simulink model "torqueControlBalancingR2022a"  (R2022a)
settings: Solver=FixedStepDiscrete  StartTime=0.0  StopTime=Config.SIMULATION_TIME  FixedStep=Config.tStep  RelTol=1e-3  EnableMultiTasking=on
PostLoadFcn:
  | %% Try to open the static GUI and try to adjust it
  | try
  | 
  |     staticGUI = simulinkStaticGUI;
  | 
  | end
InitFcn:
  | %% initialize the simulation
  | cd(fileparts(which(bdroot)));
  | initTorqueControlBalancing;
  | 
  | %% Try to edit the GUI (the user may have already closed it)
  | try
  | 
  |     %% Update Start Button
  |     set(sl_synch_handles.startButton,'Backgroundcolor',[0.0,1.0,0.0]);
  |     set(sl_synch_handles.startButton,'Enable','on');
  | 
  | end
StartFcn:
  | %% Try to edit the GUI (the user may have already closed it)
  | try
  | 
  |     %% Update Start Button
  |     set(sl_synch_handles.startButton,'Backgroundcolor',[0.8,0.8,0.8]);
  |     set(sl_synch_handles.startButton,'Enable','off');
  | 
  |     %% Update Compile Button
  |     set(sl_synch_handles.compileButton,'Backgroundcolor',[0.8,0.8,0.8]);
  |     set(sl_synch_handles.compileButton,'Enable','off');
  | 
  |     %% Update Exit Button
  |     set(sl_synch_handles.exitButton,'Backgroundcolor',[0.8,0.8,0.8]);
  |     set(sl_synch_handles.exitButton,'Enable','off');
  | 
  | end
StopFcn:
  | %% stop the simulation
  | cd(fileparts(which(bdroot)));
  | stopTorqueControlBalancing;
  | 
  | %% Try to edit the GUI (the user may have already closed it)
  | try
  | 
  |     %% Update Start Button
  |     if get(sl_synch_handles.checkbox_recompile, 'Value')
  |         set(sl_synch_handles.startButton,'Backgroundcolor',[0.0,1.0,0.0]);
  |         set(sl_synch_handles.startButton,'Enable','on');
  |     end
  | 
  |     %% Update Compile Button
  |     set(sl_synch_handles.compileButton,'Backgroundcolor',[1.0,0.6,0.0]);
  |     set(sl_synch_handles.compileButton,'Enable','on');
  | 
  |     %% Update Exit Button
  |     set(sl_synch_handles.exitButton,'Backgroundcolor',[0.0,1.0,1.0]);
  |     set(sl_synch_handles.exitButton,'Enable','on');
  | 
  | end
undefined symbols (not defined in the file or in its folder): bVectorConstraints, Config, ConstraintsMatrix, Gain, Reg, ROBOT_DOF, Sat, StateMachine
libraries: WBToolboxLibrary x57
(part 1 of 2)
CloseFcn:
  | %% Try to close the GUI (the user might have already closed it)
  | try
  | 
  |     close(simulinkStaticGUI)
  | 
  | end
settings Model: Creator=daniele  LastModifiedBy=dpucci
settings SolverCC: AlgebraicLoopSolver=TrustRegion
settings DataIOCC: LimitDataPoints=on  SaveFormat=Array  ReturnWorkspaceOutputs=off
settings OptimizationCC: ExpressionDepthLimit=2147483647  ZeroExternalMemoryAtStartup=off  ZeroInternalMemoryAtStartup=off  LifeSpan=inf
settings DebuggingCC: UnderspecifiedInitializationDetection=Classic  MergeDetectMultiDrivingBlocksExec=none  SolverPrmCheckMsg=warning  FcnCallInpInsideContextMsg=warning  UnconnectedInputMsg=warning  UnconnectedOutputMsg=warning  UnconnectedLineMsg=warning  AllowSymbolicDim=off  StateNameClashWarn=warning  SFUnexpectedBacktrackingDiag=warning  SFNoUnconditionalDefaultTransitionDiag=warning  SFExecutionAtInitializationDiag=none  ArithmeticOperatorsInVariantConditions=warning
settings HardwareCC: ProdBitPerPointer=32  ProdBitPerSizeT=32  ProdBitPerPtrDiffT=32  ProdLargestAtomicFloat=None  ProdIntDivRoundTo=Undefined  ProdEndianess=Unspecified  ProdWordSize=32  ProdHWDeviceType=32-bit Generic
settings ModelReferenceCC: PropagateSignalLabelsOutOfModel=off
settings SFSimCC: SimUseLocalCustomCode=off  SimParseCustomCode=off  CustomCodeUndefinedFunction=UseInterfaceOnly  SimTargetLang=C++
settings RTWCC: GenCodeOnly=on  RTWUseLocalCustomCode=off  TargetLang=C++
settings CodeAppCC: StateflowObjectComments=on
settings GRTTargetCC: TargetLangStandard=C++03 (ISO)  MatFileLogging=off  CodeInterfacePackaging=C++ class  SupportNonFinite=off
settings ConfigComp: CovMetricSettings=dw  CovSaveCumulativeToWorkspaceVar=on  CovSaveSingleToWorkspaceVar=on  CovExternalEMLEnable=off

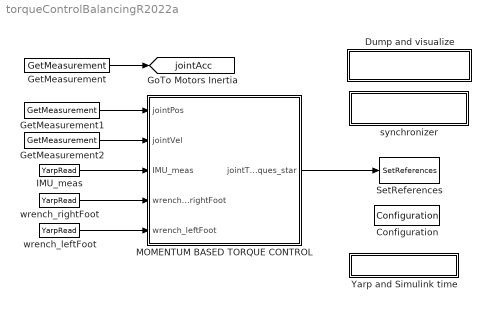
== system torqueControlBalancingR2022a ==
  " Yarp and Simulink time" : Subsystem
  Configuration : WBToolboxLibrary/Utilities/Configuration  ConfigSource=Workspace  ConfigObject='WBTConfigRobot'  RobotName='icubSim'  UrdfFile='model.urdf'  ControlledJoints={'l_elbow','l_shoulder_pitch','torso_roll'}  ControlBoardsNames={'left_arm','right_arm','torso'}  LocalName='WBT'  GravityVector=[0,0,-9.81]
      settings: SourceProductName=WholeBodyToolbox
  Dump and visualize : Subsystem
      mask Display: disp('VISUALIZER')
  GetMeasurement : WBToolboxLibrary/States/GetMeasurement  measuredType=Joints Acceleration
      settings: SourceProductName=WholeBodyToolbox
  GetMeasurement1 : WBToolboxLibrary/States/GetMeasurement  measuredType=Joints Position
      settings: SourceProductName=WholeBodyToolbox
  GetMeasurement2 : WBToolboxLibrary/States/GetMeasurement  measuredType=Joints Velocity
      settings: SourceProductName=WholeBodyToolbox
  IMU_meas : WBToolboxLibrary/Utilities/YarpRead  portName=Ports.IMU  signalSize=Ports.IMU_PORT_SIZE  timeout=0.5  blocking=off  timestamp=off  autoconnect=on  errorOnConnection=off
      settings: SourceProductName=WholeBodyToolbox
  MOMENTUM BASED TORQUE CONTROL : Subsystem
  SetReferences : WBToolboxLibrary/Actuators/SetReferences  controlType=Torque  refSpeed=50  refAcceleration=1000000*(pi/180)
      settings: SourceProductName=WholeBodyToolbox
  synchronizer : Subsystem
      mask Display: disp('SYNCHRONIZER')
  wrench_leftFoot : WBToolboxLibrary/Utilities/YarpRead  portName=Ports.WRENCH_LEFT_FOOT  signalSize=Ports.WRENCH_PORT_SIZE  timeout=0.5  blocking=off  timestamp=off  autoconnect=on  errorOnConnection=on
      settings: SourceProductName=WholeBodyToolbox
  wrench_rightFoot : WBToolboxLibrary/Utilities/YarpRead  portName=Ports.WRENCH_RIGHT_FOOT  signalSize=Ports.WRENCH_PORT_SIZE  timeout=0.5  blocking=off  timestamp=off  autoconnect=on  errorOnConnection=on
      settings: SourceProductName=WholeBodyToolbox
  tag scope: jointAcc=global
  wires:
  MOMENTUM BASED TORQUE CONTROL/1(jointTorques_star) -> SetReferences/1
  GetMeasurement/1 -> [jointAcc]
  GetMeasurement2/1 -> MOMENTUM BASED TORQUE CONTROL/2(jointVel)
  GetMeasurement1/1 -> MOMENTUM BASED TORQUE CONTROL/1(jointPos)
  IMU_meas/1 -> MOMENTUM BASED TORQUE CONTROL/3(IMU_meas)
  wrench_rightFoot/1 -> MOMENTUM BASED TORQUE CONTROL/4(wrench_rightFoot)
  wrench_leftFoot/1 -> MOMENTUM BASED TORQUE CONTROL/5(wrench_leftFoot)

== system torqueControlBalancingR2022a/ Yarp and Simulink time ==
  Clock : Clock
  Sum : Sum  Inputs=+-|
  Sum1 : Sum  Inputs=|+-
  Yarp Clock : WBToolboxLibrary/Utilities/Yarp Clock
      settings: SourceProductName=WholeBodyToolbox
  "holder " : WBToolboxLibrary/Utilities/holder 
      settings: SourceProductName=WholeBodyToolbox
  time : Scope  NumInputPorts=3
  wires:
  Yarp Clock/1 -> "holder "/1, Sum1/1  "Yarp-time"
  Sum/1 -> time/3  "Difference Simulink - Yarp time"
  Sum1/1 -> Sum/2, time/2  "Yarp-time_0"
  "holder "/1 -> Sum1/2
  Clock/1 -> Sum/1, time/1  "Simulink-time"

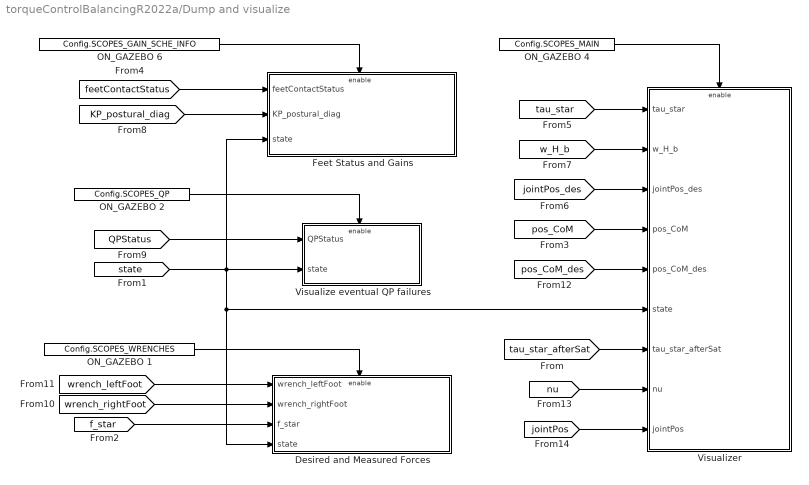
== system torqueControlBalancingR2022a/Dump and visualize ==
  Desired and Measured Forces : Subsystem
  Feet Status and Gains : Subsystem
  ON_GAZEBO 1 : Constant  Value=Config.SCOPES_WRENCHES
  ON_GAZEBO 2 : Constant  Value=Config.SCOPES_QP
  ON_GAZEBO 4 : Constant  Value=Config.SCOPES_MAIN
  ON_GAZEBO 6 : Constant  Value=Config.SCOPES_GAIN_SCHE_INFO
  Visualize eventual QP failures : Subsystem
  Visualizer : Subsystem
  wires:
  ON_GAZEBO 4/1 -> Visualizer/Enable
  [state] -> Visualize eventual QP failures/2(state), Desired and Measured Forces/4(state), Visualizer/6(state), Feet Status and Gains/3(state)
  [w_H_b] -> Visualizer/2(w_H_b)
  [tau_star] -> Visualizer/1(tau_star)
  [pos_CoM_des] -> Visualizer/5(pos_CoM_des)
  ON_GAZEBO 2/1 -> Visualize eventual QP failures/Enable
  [QPStatus] -> Visualize eventual QP failures/1(QPStatus)
  ON_GAZEBO 1/1 -> Desired and Measured Forces/Enable
  ON_GAZEBO 6/1 -> Feet Status and Gains/Enable
  [feetContactStatus] -> Feet Status and Gains/1(feetContactStatus)
  [KP_postural_diag] -> Feet Status and Gains/2(KP_postural_diag)
  [f_star] -> Desired and Measured Forces/3(f_star)
  [wrench_leftFoot] -> Desired and Measured Forces/1(wrench_leftFoot)
  [wrench_rightFoot] -> Desired and Measured Forces/2(wrench_rightFoot)
  [jointPos_des] -> Visualizer/3(jointPos_des)
  [pos_CoM] -> Visualizer/4(pos_CoM)
  [tau_star_afterSat] -> Visualizer/7(tau_star_afterSat)
  [nu] -> Visualizer/8(nu)
  [jointPos] -> Visualizer/9(jointPos)

== system torqueControlBalancingR2022a/MOMENTUM BASED TORQUE CONTROL ==
  jointPos : Inport
  jointVel : Inport  Port=2
  IMU_meas : Inport  Port=3
  wrench_rightFoot : Inport  Port=4
  wrench_leftFoot : Inport  Port=5
  Balancing Controller QP : Subsystem
  Dynamics and Kinematics : Subsystem
  Joint Torque Saturation : Subsystem
  Robot State and References : Subsystem  Priority=-10
  emergency stop: joint limits : Subsystem
      mask Display: disp('EMERGENCY STOP')
  jointTorques_star : Outport  VectorParamsAs1DForOutWhenUnconnected=off
  wires:
  Dynamics and Kinematics/4(w_H_l_sole) -> Balancing Controller QP/4(w_H_l_sole)
  Dynamics and Kinematics/11(JDot_r_sole_nu) -> Balancing Controller QP/11(JDot_r_sole_nu)
  Dynamics and Kinematics/9(pos_CoM) -> Balancing Controller QP/9(pos_CoM)
  Dynamics and Kinematics/2(h) -> Balancing Controller QP/2(h)
  Dynamics and Kinematics/8(J_CoM) -> Balancing Controller QP/8(J_CoM)
  Dynamics and Kinematics/5(w_H_r_sole) -> Balancing Controller QP/5(w_H_r_sole)
  Robot State and References/2(nu) -> Balancing Controller QP/13(nu), Dynamics and Kinematics/2(nu)
  Robot State and References/7(KD_CoM) -> Balancing Controller QP/18(KD_CoM)
  jointVel/1 -> Robot State and References/2(jointVel)
  Joint Torque Saturation/1(tau_star_sat) -> jointTorques_star/1
  Dynamics and Kinematics/7(J_r_sole) -> Balancing Controller QP/7(J_r_sole)
  Robot State and References/3(state) -> Balancing Controller QP/14(state)
  Balancing Controller QP/1("tau_star ") -> Joint Torque Saturation/1(tau_star)
  Dynamics and Kinematics/6(J_l_sole) -> Balancing Controller QP/6(J_l_sole)
  Dynamics and Kinematics/1(M) -> Balancing Controller QP/1(M)
  Robot State and References/6(KP_CoM) -> Balancing Controller QP/17(KP_CoM)
  Dynamics and Kinematics/3(L) -> Balancing Controller QP/3("L ")
  Robot State and References/9(jointPos_des) -> Balancing Controller QP/20(jointPos_des)
  Robot State and References/4(feetContactStatus) -> Balancing Controller QP/15(feetContactStatus)
  IMU_meas/1 -> Robot State and References/3(IMU_meas)
  Robot State and References/1(w_H_b) -> Dynamics and Kinematics/1(w_H_b)
  Robot State and References/5(KP_postural) -> Balancing Controller QP/16(KP_postural)
  Dynamics and Kinematics/10(JDot_l_sole_nu) -> Balancing Controller QP/10(JDot_l_sole_nu)
  Robot State and References/8(desired_pos_vel_acc_CoM) -> Balancing Controller QP/19(desired_pos_vel_acc_CoM)
  jointPos/1 -> emergency stop: joint limits/1(jointPos), Robot State and References/1(jointPos), Dynamics and Kinematics/3(jointPos), Balancing Controller QP/12(jointPos)
  wrench_rightFoot/1 -> Robot State and References/4(wrench_rightFoot)
  wrench_leftFoot/1 -> Robot State and References/5(wrench_leftFoot)

== system torqueControlBalancingR2022a/synchronizer ==
  GAZEBO_SYNCHRONIZER : Subsystem
  Logical Operator : Logic  Operator=NOT  AllPortsSameDT=off  OutDataTypeStr=boolean
  "ON_GAZEBO " : Constant  Value=Config.ON_GAZEBO
  REAL_TIME_SYNC : Subsystem
  To Workspace : ToWorkspace  VariableName=yarp_time  SaveFormat=Structure With Time  SampleTime=-1
  Yarp Clock : WBToolboxLibrary/Utilities/Yarp Clock
      settings: SourceProductName=WholeBodyToolbox
  wires:
  Logical Operator/1 -> REAL_TIME_SYNC/Enable
  "ON_GAZEBO "/1 -> GAZEBO_SYNCHRONIZER/Enable, Logical Operator/1
  Yarp Clock/1 -> To Workspace/1

== system torqueControlBalancingR2022a/Dump and visualize/Desired and Measured Forces ==
  wrench_leftFoot : Inport
  wrench_rightFoot : Inport  Port=2
  f_star : Inport  Port=3
  state : Inport  Port=4
  Enable : EnablePort
  Constant : Constant  Value=StateMachine.wrench_thresholdContactOn
  Constant2 : Constant  Value=StateMachine.wrench_thresholdContactOff
  Demux Forces nd Moments : Subsystem
  Sum{,1..3} (4 alike) : Sum  Inputs=-+|
  left Foot forces : Scope  NumInputPorts=6
  left Foot moments : Scope  NumInputPorts=4
  right Foot forces : Scope  NumInputPorts=6
  right Foot moments : Scope  NumInputPorts=4
  wires:
  wrench_leftFoot/1 -> Demux Forces nd Moments/1(wrench_leftFoot)
  wrench_rightFoot/1 -> Demux Forces nd Moments/2(wrench_rightFoot)
  f_star/1 -> Demux Forces nd Moments/3(f_star)
  Demux Forces nd Moments/1(measured forces l_sole) -> left Foot forces/1, Sum/1  "measured forces l_sole"
  Demux Forces nd Moments/2(des forces l_sole) -> Sum/2, left Foot forces/2  "desired forces l_sole"
  Sum/1 -> left Foot forces/3  "error forces l_sole"
  Constant/1 -> right Foot forces/5, left Foot forces/5  "thresholdContactOn"
  Demux Forces nd Moments/4(des forces r_sole) -> Sum1/2, right Foot forces/2  "desired forces r_sole"
  Demux Forces nd Moments/3(measured forces r_sole) -> right Foot forces/1, Sum1/1  "measured forces r_sole"
  Sum1/1 -> right Foot forces/3  "error forces r_sole"
  Constant2/1 -> left Foot forces/4, right Foot forces/4  "thresholdContactOff"
  Demux Forces nd Moments/7(measured moments r_sole) -> Sum3/1, right Foot moments/1  "measured moments r_sole"
  state/1 -> right Foot moments/4, left Foot moments/4, right Foot forces/6, left Foot forces/6  "state"
  Demux Forces nd Moments/8(des moments r_sole) -> right Foot moments/2, Sum3/2  "desired moments r_sole"
  Sum3/1 -> right Foot moments/3  "error moments r_sole"
  Sum2/1 -> left Foot moments/3  "error moments l_sole"
  Demux Forces nd Moments/6(des moments l_sole) -> Sum2/2, left Foot moments/2  "desired moments l_sole"
  Demux Forces nd Moments/5(measured moments l_sole) -> Sum2/1, left Foot moments/1  "measured moments l_sole"

== system torqueControlBalancingR2022a/Dump and visualize/Feet Status and Gains ==
  feetContactStatus : Inport
  KP_postural_diag : Inport  Port=2
  state : Inport  Port=3
  Enable : EnablePort
  Demux1 : Demux  Outputs=Config.numOfJointsForEachControlboard
  Feet Contact Activation : Scope  NumInputPorts=2
  Gain Scheduling Postural : Scope  NumInputPorts=6
  wires:
  state/1 -> Feet Contact Activation/2, Gain Scheduling Postural/6
  feetContactStatus/1 -> Feet Contact Activation/1
  KP_postural_diag/1 -> Demux1/1
  Demux1/4 -> Gain Scheduling Postural/4  "left_leg"
  Demux1/5 -> Gain Scheduling Postural/5  "right_leg"
  Demux1/3 -> Gain Scheduling Postural/3  "right_arm"
  Demux1/1 -> Gain Scheduling Postural/1  "torso"
  Demux1/2 -> Gain Scheduling Postural/2  "left_arm"

== system torqueControlBalancingR2022a/Dump and visualize/Visualize eventual QP failures ==
  QPStatus : Inport
  state : Inport  Port=2
  Enable : EnablePort
  QP status (0: no failure) : Scope  NumInputPorts=2
  wires:
  QPStatus/1 -> QP status (0: no failure)/1
  state/1 -> QP status (0: no failure)/2

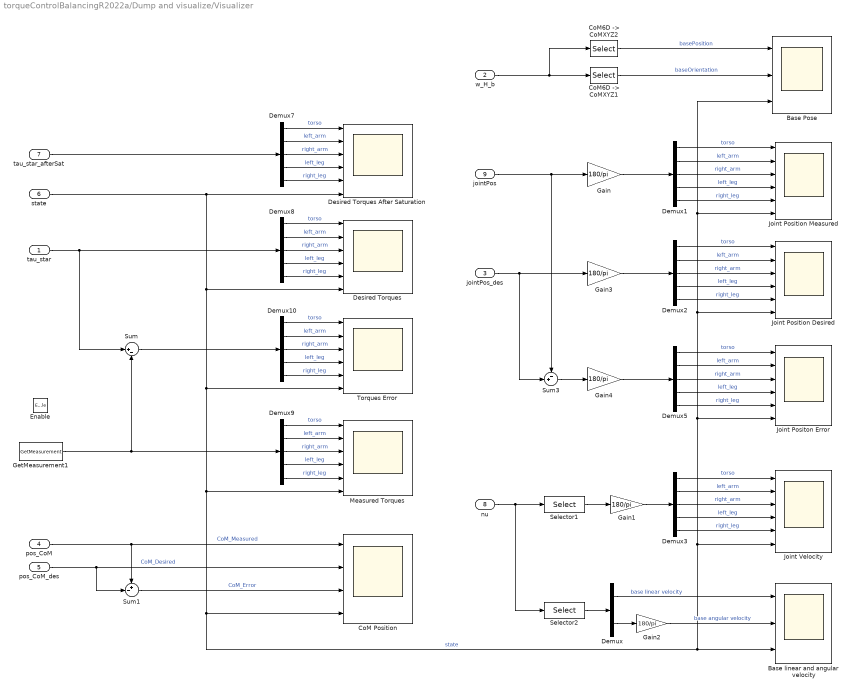
== system torqueControlBalancingR2022a/Dump and visualize/Visualizer ==
  tau_star : Inport
  w_H_b : Inport  Port=2
  jointPos_des : Inport  Port=3
  pos_CoM : Inport  Port=4
  pos_CoM_des : Inport  Port=5
  state : Inport  Port=6
  tau_star_afterSat : Inport  Port=7
  nu : Inport  Port=8
  jointPos : Inport  Port=9
  Enable : EnablePort
  Base Pose : Scope  NumInputPorts=3
  Base linear and angular velocity : Scope  NumInputPorts=3
  CoM Position : Scope  NumInputPorts=4
  "CoM6D -> CoMXYZ1" : Selector  NumberOfDimensions=2  InputPortWidth=7  IndexOptions=Index vector (dialog),Index vector (dialog)  Indices=[1 2 3],[1 2 3]  OutputSizes=1,1
  "CoM6D -> CoMXYZ2" : Selector  NumberOfDimensions=2  InputPortWidth=7  IndexOptions=Index vector (dialog),Index vector (dialog)  Indices=[1 2 3],[4]  OutputSizes=1,1
  Demux : Demux  Outputs=2
  Demux{1..3,5,7..10} (8 alike) : Demux  Outputs=Config.numOfJointsForEachControlboard
  Desired Torques : Scope  NumInputPorts=6
  Desired Torques After Saturation : Scope  NumInputPorts=6
  Gain{,1..4} (5 alike) : Gain  Gain=180/pi
  GetMeasurement1 : WBToolboxLibrary/States/GetMeasurement  measuredType=Joints Torque
      settings: SourceProductName=WholeBodyToolbox
  Joint Position Desired : Scope  NumInputPorts=6
  Joint Position Measured : Scope  NumInputPorts=6
  Joint Positon Error : Scope  NumInputPorts=6
  Joint Velocity : Scope  NumInputPorts=6
  Measured Torques : Scope  NumInputPorts=6
  Selector1 : Selector  InputPortWidth=6+ROBOT_DOF  IndexOptions=Index vector (dialog)  Indices=[7:6+ROBOT_DOF]  OutputSizes=1
  Selector2 : Selector  InputPortWidth=6+ROBOT_DOF  IndexOptions=Index vector (dialog)  Indices=[1:6]  OutputSizes=1
  Sum : Sum  Inputs=|+-
  Sum1 : Sum  Inputs=+-|
  Sum3 : Sum  Inputs=-+|
  Torques Error : Scope  NumInputPorts=6
  wires:
  pos_CoM/1 -> Sum1/1, CoM Position/1  "CoM_Measured"
  Gain/1 -> Demux1/1
  jointPos/1 -> Gain/1, Sum3/1
  Demux1/5 -> Joint Position Measured/5  "right_leg"
  Demux1/1 -> Joint Position Measured/1  "torso"
  Demux1/2 -> Joint Position Measured/2  "left_arm"
  Demux1/4 -> Joint Position Measured/4  "left_leg"
  Demux1/3 -> Joint Position Measured/3  "right_arm"
  GetMeasurement1/1 -> Sum/2, Demux9/1
  Demux8/5 -> Desired Torques/5  "right_leg"
  Demux8/1 -> Desired Torques/1  "torso"
  Demux8/2 -> Desired Torques/2  "left_arm"
  Demux8/4 -> Desired Torques/4  "left_leg"
  Demux8/3 -> Desired Torques/3  "right_arm"
  Demux10/5 -> Torques Error/5  "right_leg"
  Demux10/1 -> Torques Error/1  "torso"
  Demux10/2 -> Torques Error/2  "left_arm"
  Demux10/4 -> Torques Error/4  "left_leg"
  Demux10/3 -> Torques Error/3  "right_arm"
  Sum/1 -> Demux10/1
  Demux9/5 -> Measured Torques/5  "right_leg"
  Demux9/1 -> Measured Torques/1  "torso"
  Demux9/2 -> Measured Torques/2  "left_arm"
  Demux9/4 -> Measured Torques/4  "left_leg"
  Demux9/3 -> Measured Torques/3  "right_arm"
  jointPos_des/1 -> Sum3/2, Gain3/1
  Gain3/1 -> Demux2/1
  Demux2/5 -> Joint Position Desired/5  "right_leg"
  Demux2/1 -> Joint Position Desired/1  "torso"
  Demux2/2 -> Joint Position Desired/2  "left_arm"
  Demux2/4 -> Joint Position Desired/4  "left_leg"
  Demux2/3 -> Joint Position Desired/3  "right_arm"
  Gain4/1 -> Demux5/1
  Demux5/5 -> Joint Positon Error/5  "right_leg"
  Demux5/1 -> Joint Positon Error/1  "torso"
  Demux5/2 -> Joint Positon Error/2  "left_arm"
  Demux5/4 -> Joint Positon Error/4  "left_leg"
  Demux5/3 -> Joint Positon Error/3  "right_arm"
  Sum3/1 -> Gain4/1
  pos_CoM_des/1 -> Sum1/2, CoM Position/2  "CoM_Desired"
  w_H_b/1 -> "CoM6D -> CoMXYZ2"/1, "CoM6D -> CoMXYZ1"/1
  "CoM6D -> CoMXYZ2"/1 -> Base Pose/1  "basePosition"
  "CoM6D -> CoMXYZ1"/1 -> Base Pose/2  "baseOrientation"
  Demux7/4 -> Desired Torques After Saturation/4  "left_leg"
  Demux7/5 -> Desired Torques After Saturation/5  "right_leg"
  Demux7/2 -> Desired Torques After Saturation/2  "left_arm"
  Demux7/1 -> Desired Torques After Saturation/1  "torso"
  Demux7/3 -> Desired Torques After Saturation/3  "right_arm"
  tau_star_afterSat/1 -> Demux7/1
  tau_star/1 -> Sum/1, Demux8/1
  nu/1 -> Selector1/1, Selector2/1
  Selector2/1 -> Demux/1
  Gain1/1 -> Demux3/1
  Demux/1 -> Base linear and angular velocity/1  "base linear velocity"
  Gain2/1 -> Base linear and angular velocity/2  "base angular velocity"
  Demux3/3 -> Joint Velocity/3  "right_arm"
  Demux3/5 -> Joint Velocity/5  "right_leg"
  Selector1/1 -> Gain1/1
  Demux3/1 -> Joint Velocity/1  "torso"
  Demux3/2 -> Joint Velocity/2  "left_arm"
  Demux3/4 -> Joint Velocity/4  "left_leg"
  Demux/2 -> Gain2/1
  Sum1/1 -> CoM Position/3  "CoM_Error"
  state/1 -> Base linear and angular velocity/3, Joint Velocity/6, Joint Positon Error/6, Joint Position Desired/6, Base Pose/3, Joint Position Measured/6, CoM Position/4, Measured Torques/6, Torques Error/6, Desired Torques/6, Desired Torques After Saturation/6  "state"

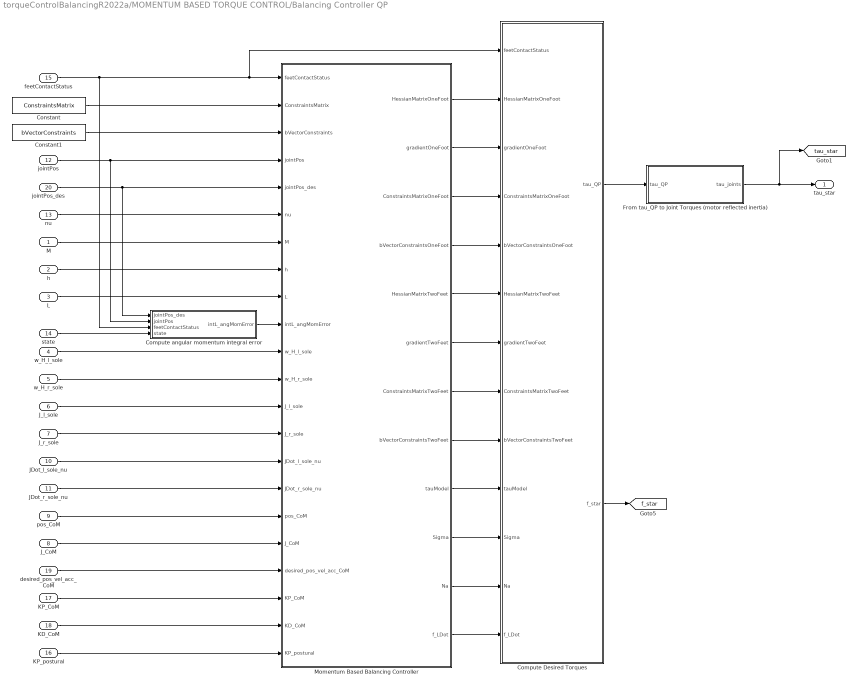
== system torqueControlBalancingR2022a/MOMENTUM BASED TORQUE CONTROL/Balancing Controller QP ==
  M : Inport
  h : Inport  Port=2
  "L " : Inport  Port=3
  w_H_l_sole : Inport  Port=4
  w_H_r_sole : Inport  Port=5
  J_l_sole : Inport  Port=6
  J_r_sole : Inport  Port=7
  J_CoM : Inport  Port=8
  pos_CoM : Inport  Port=9
  JDot_l_sole_nu : Inport  Port=10
  JDot_r_sole_nu : Inport  Port=11
  jointPos : Inport  Port=12
  nu : Inport  Port=13
  state : Inport  Port=14
  feetContactStatus : Inport  Port=15
  KP_postural : Inport  Port=16
  KP_CoM : Inport  Port=17
  KD_CoM : Inport  Port=18
  desired_pos_vel_acc_CoM : Inport  Port=19
  jointPos_des : Inport  Port=20
  Compute Desired Torques : Subsystem
  Compute angular momentum integral error : Subsystem
  Constant : Constant  Value=ConstraintsMatrix
  Constant1 : Constant  Value=bVectorConstraints
  From tau_QP to Joint Torques (motor reflected inertia) : Subsystem
  "Momentum Based Balancing Controller " : MATLAB Function  TreatAsAtomicUnit=on
  "tau_star " : Outport  VectorParamsAs1DForOutWhenUnconnected=off
  tag scope: f_star=global, tau_star=global
  wires:
  Compute Desired Torques/1(tau_QP) -> From tau_QP to Joint Torques (motor reflected inertia)/1(tau_QP)
  Compute Desired Torques/2(f_star) -> [f_star]
  From tau_QP to Joint Torques (motor reflected inertia)/1(tau_joints) -> [tau_star], "tau_star "/1
  feetContactStatus/1 -> Compute angular momentum integral error/3(feetContactStatus), "Momentum Based Balancing Controller "/1(feetContactStatus), Compute Desired Torques/1(feetContactStatus)
  Constant1/1 -> "Momentum Based Balancing Controller "/3(bVectorConstraints)
  Constant/1 -> "Momentum Based Balancing Controller "/2(ConstraintsMatrix)
  jointPos/1 -> Compute angular momentum integral error/2(jointPos), "Momentum Based Balancing Controller "/4(jointPos)
  jointPos_des/1 -> Compute angular momentum integral error/1(jointPos_des), "Momentum Based Balancing Controller "/5(jointPos_des)
  nu/1 -> "Momentum Based Balancing Controller "/6(nu)
  M/1 -> "Momentum Based Balancing Controller "/7(M)
  h/1 -> "Momentum Based Balancing Controller "/8(h)
  "L "/1 -> "Momentum Based Balancing Controller "/9(L)
  Compute angular momentum integral error/1(intL_angMomError) -> "Momentum Based Balancing Controller "/10(intL_angMomError)
  w_H_l_sole/1 -> "Momentum Based Balancing Controller "/11(w_H_l_sole)
  w_H_r_sole/1 -> "Momentum Based Balancing Controller "/12(w_H_r_sole)
  J_l_sole/1 -> "Momentum Based Balancing Controller "/13(J_l_sole)
  J_r_sole/1 -> "Momentum Based Balancing Controller "/14(J_r_sole)
  JDot_l_sole_nu/1 -> "Momentum Based Balancing Controller "/15(JDot_l_sole_nu)
  JDot_r_sole_nu/1 -> "Momentum Based Balancing Controller "/16(JDot_r_sole_nu)
  pos_CoM/1 -> "Momentum Based Balancing Controller "/17(pos_CoM)
  J_CoM/1 -> "Momentum Based Balancing Controller "/18(J_CoM)
  desired_pos_vel_acc_CoM/1 -> "Momentum Based Balancing Controller "/19(desired_pos_vel_acc_CoM)
  KP_CoM/1 -> "Momentum Based Balancing Controller "/20(KP_CoM)
  KD_CoM/1 -> "Momentum Based Balancing Controller "/21(KD_CoM)
  KP_postural/1 -> "Momentum Based Balancing Controller "/22(KP_postural)
  "Momentum Based Balancing Controller "/1(HessianMatrixOneFoot) -> Compute Desired Torques/2(HessianMatrixOneFoot)
  "Momentum Based Balancing Controller "/2(gradientOneFoot) -> Compute Desired Torques/3(gradientOneFoot)
  "Momentum Based Balancing Controller "/3(ConstraintsMatrixOneFoot) -> Compute Desired Torques/4(ConstraintsMatrixOneFoot)
  "Momentum Based Balancing Controller "/4(bVectorConstraintsOneFoot) -> Compute Desired Torques/5(bVectorConstraintsOneFoot)
  "Momentum Based Balancing Controller "/5(HessianMatrixTwoFeet) -> Compute Desired Torques/6(HessianMatrixTwoFeet)
  "Momentum Based Balancing Controller "/6(gradientTwoFeet) -> Compute Desired Torques/7(gradientTwoFeet)
  "Momentum Based Balancing Controller "/7(ConstraintsMatrixTwoFeet) -> Compute Desired Torques/8(ConstraintsMatrixTwoFeet)
  "Momentum Based Balancing Controller "/8(bVectorConstraintsTwoFeet) -> Compute Desired Torques/9(bVectorConstraintsTwoFeet)
  "Momentum Based Balancing Controller "/9(tauModel) -> Compute Desired Torques/10(tauModel)
  "Momentum Based Balancing Controller "/10(Sigma) -> Compute Desired Torques/11(Sigma)
  "Momentum Based Balancing Controller "/11(Na) -> Compute Desired Torques/12(Na)
  "Momentum Based Balancing Controller "/12(f_LDot) -> Compute Desired Torques/13(f_LDot)
  state/1 -> Compute angular momentum integral error/4(state)

== system torqueControlBalancingR2022a/MOMENTUM BASED TORQUE CONTROL/Dynamics and Kinematics ==
  w_H_b : Inport
  nu : Inport  Port=2
  jointPos : Inport  Port=3
  Dynamics : Subsystem
  Kinematics : Subsystem
  M : Outport  VectorParamsAs1DForOutWhenUnconnected=off
  h : Outport  Port=2  VectorParamsAs1DForOutWhenUnconnected=off
  L : Outport  Port=3  VectorParamsAs1DForOutWhenUnconnected=off
  w_H_l_sole : Outport  Port=4  VectorParamsAs1DForOutWhenUnconnected=off
  w_H_r_sole : Outport  Port=5  VectorParamsAs1DForOutWhenUnconnected=off
  J_l_sole : Outport  Port=6  VectorParamsAs1DForOutWhenUnconnected=off
  J_r_sole : Outport  Port=7  VectorParamsAs1DForOutWhenUnconnected=off
  J_CoM : Outport  Port=8  VectorParamsAs1DForOutWhenUnconnected=off
  pos_CoM : Outport  Port=9  VectorParamsAs1DForOutWhenUnconnected=off
  JDot_l_sole_nu : Outport  Port=10  VectorParamsAs1DForOutWhenUnconnected=off
  JDot_r_sole_nu : Outport  Port=11  VectorParamsAs1DForOutWhenUnconnected=off
  wires:
  w_H_b/1 -> Kinematics/3(w_H_b), Dynamics/1(w_H_b)
  jointPos/1 -> Dynamics/2(jointPos), Kinematics/2(jointPos)
  nu/1 -> Dynamics/3(nu), Kinematics/1(nu)
  Dynamics/1(M) -> M/1
  Dynamics/2(h) -> h/1
  Dynamics/3(L) -> L/1
  Kinematics/7(JDot_l_sole_nu) -> JDot_l_sole_nu/1
  Kinematics/8(JDot_r_sole_nu) -> JDot_r_sole_nu/1
  Kinematics/4(J_r_sole) -> J_r_sole/1
  Kinematics/1(w_H_l_sole) -> w_H_l_sole/1
  Kinematics/3(J_l_sole) -> J_l_sole/1
  Kinematics/5(J_CoM) -> J_CoM/1
  Kinematics/6(pos_CoM) -> pos_CoM/1
  Kinematics/2(w_H_r_sole) -> w_H_r_sole/1

== system torqueControlBalancingR2022a/MOMENTUM BASED TORQUE CONTROL/Joint Torque Saturation ==
  tau_star : Inport
  Constant : Constant  Value=Config.SATURATE_TORQUE_DERIVATIVE
  Constant1 : Constant  Value=Config.tStep
  Constant2 : Constant  Value=Sat.uDotMax
  Saturate Torque Derivative : MATLAB Function  TreatAsAtomicUnit=on
  Saturation : Saturate  UpperLimit=Sat.torque  LowerLimit=-Sat.torque
  Switch : Switch  Criteria=u2 > Threshold  SaturateOnIntegerOverflow=off  InputSameDT=off
  "holder " : WBToolboxLibrary/Utilities/holder 
      settings: SourceProductName=WholeBodyToolbox
  tau_star_sat : Outport  VectorParamsAs1DForOutWhenUnconnected=off
  tag scope: tau_star_afterSat=global
  wires:
  Switch/1 -> Saturation/1
  Constant/1 -> Switch/2
  tau_star/1 -> Switch/3, Saturate Torque Derivative/1(u), "holder "/1
  Saturate Torque Derivative/1(uSat) -> Switch/1
  "holder "/1 -> Saturate Torque Derivative/2(u_0)
  Saturation/1 -> [tau_star_afterSat], tau_star_sat/1
  Constant1/1 -> Saturate Torque Derivative/3(tStep)
  Constant2/1 -> Saturate Torque Derivative/4(uDotMax)

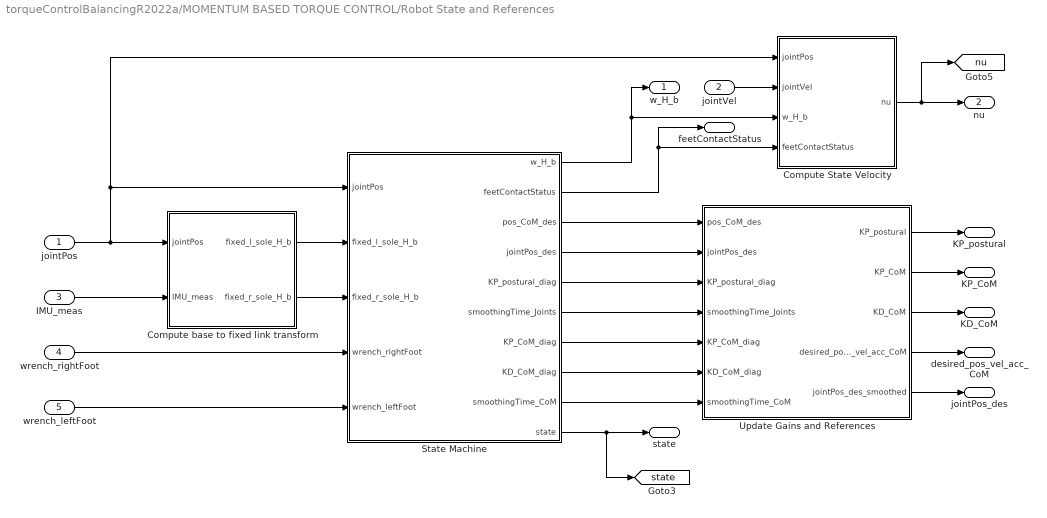
== system torqueControlBalancingR2022a/MOMENTUM BASED TORQUE CONTROL/Robot State and References ==
  jointPos : Inport
  jointVel : Inport  Port=2
  IMU_meas : Inport  Port=3
  wrench_rightFoot : Inport  Port=4
  wrench_leftFoot : Inport  Port=5
  Compute State Velocity : Subsystem
  Compute base to fixed link transform : Subsystem
  State Machine : Subsystem  Priority=-100
  Update Gains and References : Subsystem
  w_H_b : Outport  VectorParamsAs1DForOutWhenUnconnected=off
  nu : Outport  Port=2  VectorParamsAs1DForOutWhenUnconnected=off
  state : Outport  Port=3  VectorParamsAs1DForOutWhenUnconnected=off
  feetContactStatus : Outport  Port=4  VectorParamsAs1DForOutWhenUnconnected=off
  KP_postural : Outport  Port=5  VectorParamsAs1DForOutWhenUnconnected=off
  KP_CoM : Outport  Port=6  VectorParamsAs1DForOutWhenUnconnected=off
  KD_CoM : Outport  Port=7  VectorParamsAs1DForOutWhenUnconnected=off
  desired_pos_vel_acc_CoM : Outport  Port=8  VectorParamsAs1DForOutWhenUnconnected=off
  jointPos_des : Outport  Port=9  VectorParamsAs1DForOutWhenUnconnected=off
  tag scope: nu=global, state=global
  wires:
  Compute base to fixed link transform/1(fixed_l_sole_H_b) -> State Machine/2(fixed_l_sole_H_b)
  Compute base to fixed link transform/2(fixed_r_sole_H_b) -> State Machine/3(fixed_r_sole_H_b)
  State Machine/1(w_H_b) -> Compute State Velocity/3(w_H_b), w_H_b/1
  State Machine/2(feetContactStatus) -> Compute State Velocity/4("feetContactStatus "), feetContactStatus/1
  State Machine/3(pos_CoM_des) -> Update Gains and References/1(pos_CoM_des)
  State Machine/4(jointPos_des) -> Update Gains and References/2(jointPos_des)
  State Machine/5(KP_postural_diag) -> Update Gains and References/3(KP_postural_diag)
  State Machine/6(smoothingTime_Joints) -> Update Gains and References/4(smoothingTime_Joints)
  State Machine/7(KP_CoM_diag) -> Update Gains and References/5(KP_CoM_diag)
  State Machine/8(KD_CoM_diag) -> Update Gains and References/6(KD_CoM_diag)
  State Machine/9(smoothingTime_CoM) -> Update Gains and References/7(smoothingTime_CoM)
  State Machine/10(state) -> [state], state/1
  Compute State Velocity/1(nu) -> [nu], nu/1
  Update Gains and References/1(KP_postural) -> KP_postural/1
  Update Gains and References/2(KP_CoM) -> KP_CoM/1
  Update Gains and References/3(KD_CoM) -> KD_CoM/1
  Update Gains and References/4(desired_pos_vel_acc_CoM) -> desired_pos_vel_acc_CoM/1
  Update Gains and References/5(jointPos_des_smoothed) -> jointPos_des/1
  IMU_meas/1 -> Compute base to fixed link transform/2(IMU_meas)
  jointPos/1 -> Compute State Velocity/1(jointPos), State Machine/1(jointPos), Compute base to fixed link transform/1(jointPos)
  wrench_leftFoot/1 -> State Machine/5(wrench_leftFoot)
  wrench_rightFoot/1 -> State Machine/4(wrench_rightFoot)
  jointVel/1 -> Compute State Velocity/2(jointVel)

== system torqueControlBalancingR2022a/MOMENTUM BASED TORQUE CONTROL/emergency stop: joint limits ==
  jointPos : Inport
  ON_GAZEBO 1 : Constant  Value=Config.EMERGENCY_STOP_WITH_JOINTS_LIMITS
  ON_GAZEBO 2 : Constant  Value=Config.EMERGENCY_STOP_WITH_ENCODER_SPIKES
  STOP IF JOINTS HIT THE LIMITS : Subsystem
  STOP IF THERE ARE SPIKES IN THE ENCODERS : Subsystem
  wires:
  ON_GAZEBO 1/1 -> STOP IF JOINTS HIT THE LIMITS/Enable
  jointPos/1 -> STOP IF THERE ARE SPIKES IN THE ENCODERS/1(jointPos), STOP IF JOINTS HIT THE LIMITS/1(jointPos)
  ON_GAZEBO 2/1 -> STOP IF THERE ARE SPIKES IN THE ENCODERS/Enable

== system torqueControlBalancingR2022a/synchronizer/GAZEBO_SYNCHRONIZER ==
  Enable : EnablePort
  Simulator Synchronizer : WBToolboxLibrary/Utilities/Simulator Synchronizer  period=Config.tStep  serverPortName='/clock/rpc'  clientPortName='/WBT_synchronizer/rpc:o'
      settings: SourceProductName=WholeBodyToolbox

== system torqueControlBalancingR2022a/synchronizer/REAL_TIME_SYNC ==
  Enable : EnablePort
  Real Time Synchronizer : WBToolboxLibrary/Utilities/Real Time Synchronizer  period=Config.tStep
      settings: SourceProductName=WholeBodyToolbox

== system torqueControlBalancingR2022a/Dump and visualize/Desired and Measured Forces/Demux Forces nd Moments ==
  wrench_leftFoot : Inport
  wrench_rightFoot : Inport  Port=2
  f_star : Inport  Port=3
  Demux{1,5..7} (4 alike) : Demux  Outputs=[3;3]
  Demux2 : Demux  Outputs=[6;6]
  measured forces l_sole : Outport  VectorParamsAs1DForOutWhenUnconnected=off
  des forces l_sole : Outport  Port=2  VectorParamsAs1DForOutWhenUnconnected=off
  measured forces r_sole : Outport  Port=3  VectorParamsAs1DForOutWhenUnconnected=off
  des forces r_sole : Outport  Port=4  VectorParamsAs1DForOutWhenUnconnected=off
  measured moments l_sole : Outport  Port=5  VectorParamsAs1DForOutWhenUnconnected=off
  des moments l_sole : Outport  Port=6  VectorParamsAs1DForOutWhenUnconnected=off
  measured moments r_sole : Outport  Port=7  VectorParamsAs1DForOutWhenUnconnected=off
  des moments r_sole : Outport  Port=8  VectorParamsAs1DForOutWhenUnconnected=off
  wires:
  Demux6/2 -> des moments r_sole/1
  Demux5/2 -> des moments l_sole/1
  Demux1/1 -> measured forces l_sole/1
  Demux7/1 -> measured forces r_sole/1
  Demux7/2 -> measured moments r_sole/1
  wrench_leftFoot/1 -> Demux1/1
  Demux2/1 -> Demux5/1
  wrench_rightFoot/1 -> Demux7/1
  Demux6/1 -> des forces r_sole/1
  Demux1/2 -> measured moments l_sole/1
  f_star/1 -> Demux2/1
  Demux2/2 -> Demux6/1
  Demux5/1 -> des forces l_sole/1

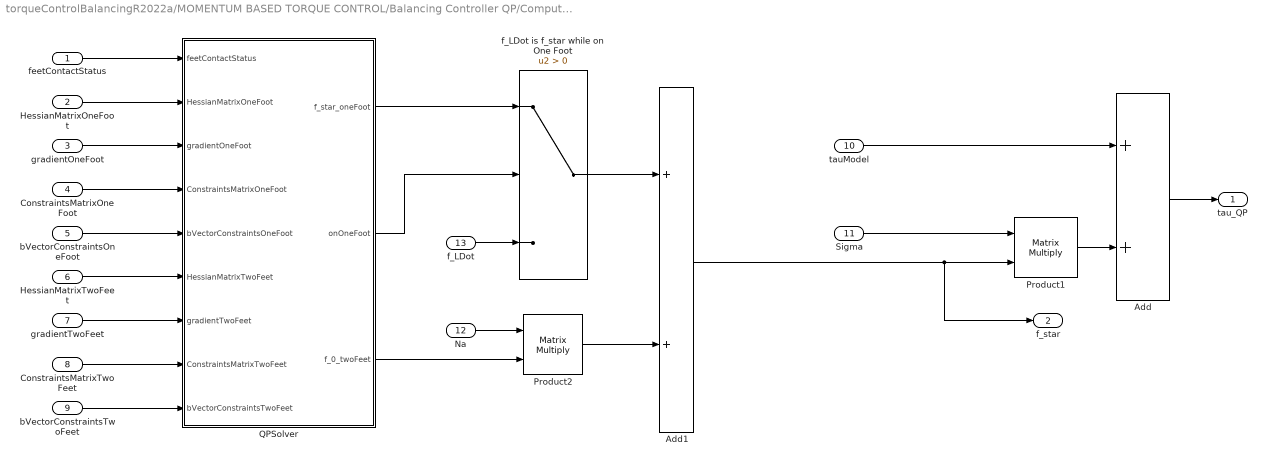
== system torqueControlBalancingR2022a/MOMENTUM BASED TORQUE CONTROL/Balancing Controller QP/Compute Desired Torques ==
  feetContactStatus : Inport
  HessianMatrixOneFoot : Inport  Port=2
  gradientOneFoot : Inport  Port=3
  ConstraintsMatrixOneFoot : Inport  Port=4
  bVectorConstraintsOneFoot : Inport  Port=5
  HessianMatrixTwoFeet : Inport  Port=6
  gradientTwoFeet : Inport  Port=7
  ConstraintsMatrixTwoFeet : Inport  Port=8
  bVectorConstraintsTwoFeet : Inport  Port=9
  tauModel : Inport  Port=10
  Sigma : Inport  Port=11
  Na : Inport  Port=12
  f_LDot : Inport  Port=13
  Add : Sum
  Add1 : Sum
  Product1 : Product  Multiplication=Matrix(*)
  Product2 : Product  Multiplication=Matrix(*)
  QPSolver : Subsystem
  f_LDot is f_star while on One Foot : Switch  Criteria=u2 > Threshold  SaturateOnIntegerOverflow=off  InputSameDT=off
  tau_QP : Outport  VectorParamsAs1DForOutWhenUnconnected=off
  f_star : Outport  Port=2  VectorParamsAs1DForOutWhenUnconnected=off
  wires:
  Na/1 -> Product2/1
  Product1/1 -> Add/2
  tauModel/1 -> Add/1
  Add/1 -> tau_QP/1
  Add1/1 -> f_star/1, Product1/2
  f_LDot is f_star while on One Foot/1 -> Add1/1
  Product2/1 -> Add1/2
  Sigma/1 -> Product1/1
  QPSolver/3(f_0_twoFeet) -> Product2/2
  gradientOneFoot/1 -> QPSolver/3(gradientOneFoot)
  ConstraintsMatrixTwoFeet/1 -> QPSolver/8(ConstraintsMatrixTwoFeet)
  feetContactStatus/1 -> QPSolver/1(feetContactStatus)
  bVectorConstraintsOneFoot/1 -> QPSolver/5(bVectorConstraintsOneFoot)
  HessianMatrixOneFoot/1 -> QPSolver/2(HessianMatrixOneFoot)
  ConstraintsMatrixOneFoot/1 -> QPSolver/4(ConstraintsMatrixOneFoot)
  gradientTwoFeet/1 -> QPSolver/7(gradientTwoFeet)
  HessianMatrixTwoFeet/1 -> QPSolver/6(HessianMatrixTwoFeet)
  bVectorConstraintsTwoFeet/1 -> QPSolver/9(bVectorConstraintsTwoFeet)
  QPSolver/2(onOneFoot) -> f_LDot is f_star while on One Foot/2
  f_LDot/1 -> f_LDot is f_star while on One Foot/3
  QPSolver/1(f_star_oneFoot) -> f_LDot is f_star while on One Foot/1

== system torqueControlBalancingR2022a/MOMENTUM BASED TORQUE CONTROL/Balancing Controller QP/Compute angular momentum integral error ==
  jointPos_des : Inport
  jointPos : Inport  Port=2
  feetContactStatus : Inport  Port=3
  state : Inport  Port=4
  Add : Sum  Inputs=-+
  CentroidalMomentum : WBToolboxLibrary/Model/Dynamics/CentroidalMomentum
      settings: SourceProductName=WholeBodyToolbox
  Compute base to fixed link transform : Subsystem
  Get Equivalent Base Velocity : MATLAB Function  TreatAsAtomicUnit=on
  Jacobian : WBToolboxLibrary/Model/Jacobians/Jacobian  frameName=Frames.LEFT_FOOT
      settings: SourceProductName=WholeBodyToolbox
  Jacobian1 : WBToolboxLibrary/Model/Jacobians/Jacobian  frameName=Frames.RIGHT_FOOT
      settings: SourceProductName=WholeBodyToolbox
  Select base to world transform : MATLAB Function  TreatAsAtomicUnit=on
  Selector : Selector  InputPortWidth=6  IndexOptions=Index vector (dialog)  Indices=[4 5 6]  OutputSizes=1
  Switch : Switch  Criteria=u2 > Threshold  Threshold=0.1  SaturateOnIntegerOverflow=off  InputSameDT=off
  intL_angMomError : Outport  VectorParamsAs1DForOutWhenUnconnected=off
  wires:
  jointPos_des/1 -> Add/1, Jacobian1/2, Jacobian/2, CentroidalMomentum/2, Compute base to fixed link transform/1(jointPos)
  jointPos/1 -> Add/2
  Add/1 -> Get Equivalent Base Velocity/4(jointPos_err), CentroidalMomentum/4
  Get Equivalent Base Velocity/1(baseVel_equivalent) -> CentroidalMomentum/3
  CentroidalMomentum/1 -> Selector/1
  Selector/1 -> intL_angMomError/1
  state/1 -> Select base to world transform/1(state)
  Select base to world transform/1(booleanState) -> Switch/2
  Switch/1 -> CentroidalMomentum/1, Jacobian/1, Jacobian1/1
  Compute base to fixed link transform/1(fixed_l_sole_H_b) -> Switch/1
  Compute base to fixed link transform/2(fixed_r_sole_H_b) -> Switch/3
  Jacobian/1 -> Get Equivalent Base Velocity/1(J_l_sole)
  Jacobian1/1 -> Get Equivalent Base Velocity/2(J_r_sole)
  feetContactStatus/1 -> Get Equivalent Base Velocity/3(feetContactStatus)

== system torqueControlBalancingR2022a/MOMENTUM BASED TORQUE CONTROL/Balancing Controller QP/From tau_QP to Joint Torques (motor reflected inertia) ==
  tau_QP : Inport
  " " : Constant  Value=Config.USE_MOTOR_REFLECTED_INERTIA
  " 1" : Constant  Value=Config.USE_DES_JOINT_ACC_FOR_MOTORS_INERTIA
  "(transpose(T*Gamma))^{-1}*I_m*(T*Gamma)^{-1}" : MATLAB Function  TreatAsAtomicUnit=on
  Add : Sum  Inputs=-+
  Gain : Gain  Gain=Config.K_ff
  Product : Product  Multiplication=Matrix(*)
  Switch : Switch  Criteria=u2 > Threshold  SaturateOnIntegerOverflow=off  InputSameDT=off
  Switch1 : Switch  Criteria=u2 > Threshold  SaturateOnIntegerOverflow=off  InputSameDT=off
  tau_joints : Outport  VectorParamsAs1DForOutWhenUnconnected=off
  wires:
  Product/1 -> Gain/1
  Gain/1 -> Add/1
  Add/1 -> Switch/1
  " "/1 -> Switch/2
  Switch/1 -> tau_joints/1
  tau_QP/1 -> Add/2, Switch/3
  "(transpose(T*Gamma))^{-1}*I_m*(T*Gamma)^{-1}"/1(reflectedInertia) -> Product/1
  " 1"/1 -> Switch1/2
  Switch1/1 -> Product/2
  [jointAcc_des] -> Switch1/1
  [jointAcc] -> Switch1/3

== system torqueControlBalancingR2022a/MOMENTUM BASED TORQUE CONTROL/Dynamics and Kinematics/Dynamics ==
  w_H_b : Inport
  jointPos : Inport  Port=2
  nu : Inport  Port=3
  Add motors reflected inertia : Subsystem
  CentroidalMomentum : WBToolboxLibrary/Model/Dynamics/CentroidalMomentum
      settings: SourceProductName=WholeBodyToolbox
  "CoM6D -> CoMXYZ1" : Selector  InputPortWidth=6+ROBOT_DOF  IndexOptions=Index vector (dialog)  Indices=[7:6+ROBOT_DOF]  OutputSizes=1
  "CoM6D -> CoMXYZ2" : Selector  InputPortWidth=6+ROBOT_DOF  IndexOptions=Index vector (dialog)  Indices=[1 2 3 4 5 6]  OutputSizes=1
  GetBiasForces : WBToolboxLibrary/Model/Dynamics/GetBiasForces
      settings: SourceProductName=WholeBodyToolbox
  MassMatrix : WBToolboxLibrary/Model/Dynamics/MassMatrix
      settings: SourceProductName=WholeBodyToolbox
  M : Outport  VectorParamsAs1DForOutWhenUnconnected=off
  h : Outport  Port=2  VectorParamsAs1DForOutWhenUnconnected=off
  L : Outport  Port=3  VectorParamsAs1DForOutWhenUnconnected=off
  wires:
  CentroidalMomentum/1 -> L/1
  GetBiasForces/1 -> h/1
  w_H_b/1 -> CentroidalMomentum/1, GetBiasForces/1, MassMatrix/1
  jointPos/1 -> CentroidalMomentum/2, GetBiasForces/2, MassMatrix/2
  "CoM6D -> CoMXYZ2"/1 -> CentroidalMomentum/3, GetBiasForces/3
  "CoM6D -> CoMXYZ1"/1 -> CentroidalMomentum/4, GetBiasForces/4
  nu/1 -> "CoM6D -> CoMXYZ1"/1, "CoM6D -> CoMXYZ2"/1
  MassMatrix/1 -> Add motors reflected inertia/1(M)
  Add motors reflected inertia/1(M_with_motor_inertia) -> M/1

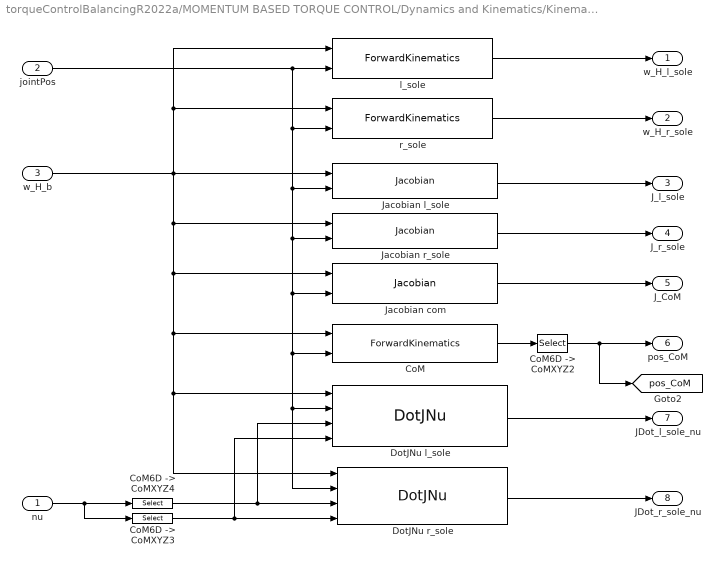
== system torqueControlBalancingR2022a/MOMENTUM BASED TORQUE CONTROL/Dynamics and Kinematics/Kinematics ==
  nu : Inport
  jointPos : Inport  Port=2
  w_H_b : Inport  Port=3
  CoM : WBToolboxLibrary/Model/Kinematics/ForwardKinematics  frameName=Frames.COM
      settings: SourceProductName=WholeBodyToolbox
  "CoM6D -> CoMXYZ2" : Selector  NumberOfDimensions=2  InputPortWidth=7  IndexOptions=Index vector (dialog),Index vector (dialog)  Indices=[1 2 3],[4]  OutputSizes=1,1
  "CoM6D -> CoMXYZ3" : Selector  InputPortWidth=6+ROBOT_DOF  IndexOptions=Index vector (dialog)  Indices=[7:6+ROBOT_DOF]  OutputSizes=1
  "CoM6D -> CoMXYZ4" : Selector  InputPortWidth=6+ROBOT_DOF  IndexOptions=Index vector (dialog)  Indices=[1 2 3 4 5 6]  OutputSizes=1
  DotJNu l_sole : WBToolboxLibrary/Model/Jacobians/DotJNu  frameName=Frames.LEFT_FOOT
      settings: SourceProductName=WholeBodyToolbox
  DotJNu r_sole : WBToolboxLibrary/Model/Jacobians/DotJNu  frameName=Frames.RIGHT_FOOT
      settings: SourceProductName=WholeBodyToolbox
  Jacobian com : WBToolboxLibrary/Model/Jacobians/Jacobian  frameName=Frames.COM
      settings: SourceProductName=WholeBodyToolbox
  Jacobian l_sole : WBToolboxLibrary/Model/Jacobians/Jacobian  frameName=Frames.LEFT_FOOT
      settings: SourceProductName=WholeBodyToolbox
  Jacobian r_sole : WBToolboxLibrary/Model/Jacobians/Jacobian  frameName=Frames.RIGHT_FOOT
      settings: SourceProductName=WholeBodyToolbox
  l_sole : WBToolboxLibrary/Model/Kinematics/ForwardKinematics  frameName=Frames.LEFT_FOOT
      settings: SourceProductName=WholeBodyToolbox
  r_sole : WBToolboxLibrary/Model/Kinematics/ForwardKinematics  frameName=Frames.RIGHT_FOOT
      settings: SourceProductName=WholeBodyToolbox
  w_H_l_sole : Outport  VectorParamsAs1DForOutWhenUnconnected=off
  w_H_r_sole : Outport  Port=2  VectorParamsAs1DForOutWhenUnconnected=off
  J_l_sole : Outport  Port=3  VectorParamsAs1DForOutWhenUnconnected=off
  J_r_sole : Outport  Port=4  VectorParamsAs1DForOutWhenUnconnected=off
  J_CoM : Outport  Port=5  VectorParamsAs1DForOutWhenUnconnected=off
  pos_CoM : Outport  Port=6  VectorParamsAs1DForOutWhenUnconnected=off
  JDot_l_sole_nu : Outport  Port=7  VectorParamsAs1DForOutWhenUnconnected=off
  JDot_r_sole_nu : Outport  Port=8  VectorParamsAs1DForOutWhenUnconnected=off
  tag scope: pos_CoM=global
  wires:
  "CoM6D -> CoMXYZ3"/1 -> DotJNu r_sole/4, DotJNu l_sole/4
  "CoM6D -> CoMXYZ4"/1 -> DotJNu r_sole/3, DotJNu l_sole/3
  nu/1 -> "CoM6D -> CoMXYZ3"/1, "CoM6D -> CoMXYZ4"/1
  l_sole/1 -> w_H_l_sole/1
  r_sole/1 -> w_H_r_sole/1
  Jacobian l_sole/1 -> J_l_sole/1
  Jacobian r_sole/1 -> J_r_sole/1
  Jacobian com/1 -> J_CoM/1
  CoM/1 -> "CoM6D -> CoMXYZ2"/1
  DotJNu l_sole/1 -> JDot_l_sole_nu/1
  DotJNu r_sole/1 -> JDot_r_sole_nu/1
  jointPos/1 -> Jacobian com/2, DotJNu r_sole/2, DotJNu l_sole/2, CoM/2, Jacobian r_sole/2, Jacobian l_sole/2, r_sole/2, l_sole/2
  w_H_b/1 -> Jacobian com/1, DotJNu r_sole/1, DotJNu l_sole/1, CoM/1, Jacobian r_sole/1, Jacobian l_sole/1, r_sole/1, l_sole/1
  "CoM6D -> CoMXYZ2"/1 -> [pos_CoM], pos_CoM/1

== system torqueControlBalancingR2022a/MOMENTUM BASED TORQUE CONTROL/Robot State and References/Compute State Velocity ==
  jointPos : Inport
  jointVel : Inport  Port=2
  w_H_b : Inport  Port=3
  "feetContactStatus " : Inport  Port=4
  Compute Base Velocity : MATLAB Function  TreatAsAtomicUnit=on
  Feet Jacobians : Subsystem
  Mux : Mux  Inputs=2
  nu : Outport  VectorParamsAs1DForOutWhenUnconnected=off
  wires:
  jointVel/1 -> Mux/2, Compute Base Velocity/4(jointVel)
  Mux/1 -> nu/1
  "feetContactStatus "/1 -> Compute Base Velocity/3(feetContactStatus)
  Compute Base Velocity/1(nu_b) -> Mux/1
  jointPos/1 -> Feet Jacobians/1(jointPos)
  w_H_b/1 -> Feet Jacobians/2(w_H_b)
  Feet Jacobians/1(J_l_sole) -> Compute Base Velocity/1(J_l_sole)
  Feet Jacobians/2(J_r_sole) -> Compute Base Velocity/2(J_r_sole)

== system torqueControlBalancingR2022a/MOMENTUM BASED TORQUE CONTROL/Robot State and References/Compute base to fixed link transform ==
  jointPos : Inport
  IMU_meas : Inport  Port=2
  Constant7 : Constant  Value=eye(4)
  "LFoot to base link transform " : Subsystem
  RFoot to base link transform : Subsystem
  Relative transform l_sole_H_base : WBToolboxLibrary/Model/Kinematics/ForwardKinematics  frameName=Frames.LEFT_FOOT
      settings: SourceProductName=WholeBodyToolbox
  Relative transform r_sole_H_base : WBToolboxLibrary/Model/Kinematics/ForwardKinematics  frameName=Frames.RIGHT_FOOT
      settings: SourceProductName=WholeBodyToolbox
  fixed_l_sole_H_b : Outport  VectorParamsAs1DForOutWhenUnconnected=off
  fixed_r_sole_H_b : Outport  Port=2  VectorParamsAs1DForOutWhenUnconnected=off
  tag scope: jointPos=global
  wires:
  Constant7/1 -> RFoot to base link transform/4(w_H_base_fixed), "LFoot to base link transform "/4(w_H_base_fixed), Relative transform r_sole_H_base/1, Relative transform l_sole_H_base/1
  RFoot to base link transform/1(link_H_b) -> fixed_r_sole_H_b/1
  "LFoot to base link transform "/1(link_H_b) -> fixed_l_sole_H_b/1
  Relative transform l_sole_H_base/1 -> "LFoot to base link transform "/3(w_H_link)
  Relative transform r_sole_H_base/1 -> RFoot to base link transform/3(w_H_link)
  jointPos/1 -> [jointPos], RFoot to base link transform/1(jointPos), "LFoot to base link transform "/1(jointPos), Relative transform r_sole_H_base/2, Relative transform l_sole_H_base/2
  IMU_meas/1 -> RFoot to base link transform/2(inertial), "LFoot to base link transform "/2(inertial)

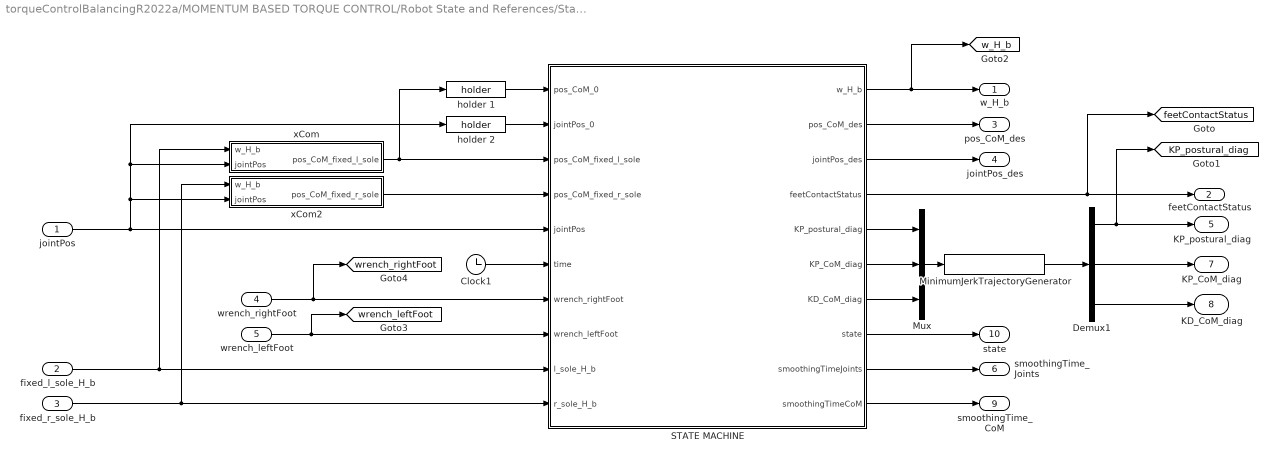
== system torqueControlBalancingR2022a/MOMENTUM BASED TORQUE CONTROL/Robot State and References/State Machine ==
  jointPos : Inport
  fixed_l_sole_H_b : Inport  Port=2
  fixed_r_sole_H_b : Inport  Port=3
  wrench_rightFoot : Inport  Port=4
  wrench_leftFoot : Inport  Port=5
  Clock1 : Clock
  Demux1 : Demux  Outputs=[ROBOT_DOF,3,3]
  MinimumJerkTrajectoryGenerator : WBToolboxLibrary/Utilities/MinimumJerkTrajectoryGenerator  externalSettlingTime=off  settlingTime=Config.SmoothingTimeGainScheduling  sampleTime=Config.tStep  resetOnSettlingTime=off  firstDerivatives=off  secondDerivatives=off  explicitInitialValue=off
      settings: SourceProductName=WholeBodyToolbox
  Mux : Mux  Inputs=3
  STATE MACHINE : MATLAB Function  TreatAsAtomicUnit=on
  holder 1 : WBToolboxLibrary/Utilities/holder 
      settings: SourceProductName=WholeBodyToolbox
  holder 2 : WBToolboxLibrary/Utilities/holder 
      settings: SourceProductName=WholeBodyToolbox
  xCom : Subsystem
  xCom2 : Subsystem
  w_H_b : Outport  VectorParamsAs1DForOutWhenUnconnected=off
  feetContactStatus : Outport  Port=2  VectorParamsAs1DForOutWhenUnconnected=off
  pos_CoM_des : Outport  Port=3  VectorParamsAs1DForOutWhenUnconnected=off
  jointPos_des : Outport  Port=4  VectorParamsAs1DForOutWhenUnconnected=off
  KP_postural_diag : Outport  Port=5  VectorParamsAs1DForOutWhenUnconnected=off
  smoothingTime_Joints : Outport  Port=6  VectorParamsAs1DForOutWhenUnconnected=off
  KP_CoM_diag : Outport  Port=7  VectorParamsAs1DForOutWhenUnconnected=off
  KD_CoM_diag : Outport  Port=8  VectorParamsAs1DForOutWhenUnconnected=off
  smoothingTime_CoM : Outport  Port=9  VectorParamsAs1DForOutWhenUnconnected=off
  state : Outport  Port=10  VectorParamsAs1DForOutWhenUnconnected=off
  tag scope: KP_postural_diag=global, feetContactStatus=global, w_H_b=global, wrench_leftFoot=global, wrench_rightFoot=global
  wires:
  xCom/1("pos_CoM_fixed_l_sole ") -> holder 1/1, STATE MACHINE/3(pos_CoM_fixed_l_sole)
  STATE MACHINE/3(jointPos_des) -> jointPos_des/1
  STATE MACHINE/2(pos_CoM_des) -> pos_CoM_des/1
  STATE MACHINE/8(state) -> state/1
  STATE MACHINE/4(feetContactStatus) -> feetContactStatus/1, [feetContactStatus]
  STATE MACHINE/9(smoothingTimeJoints) -> smoothingTime_Joints/1
  STATE MACHINE/6(KP_CoM_diag) -> Mux/2
  Demux1/3 -> KD_CoM_diag/1
  STATE MACHINE/7(KD_CoM_diag) -> Mux/3
  STATE MACHINE/5(KP_postural_diag) -> Mux/1
  Mux/1 -> MinimumJerkTrajectoryGenerator/1
  MinimumJerkTrajectoryGenerator/1 -> Demux1/1
  Demux1/1 -> [KP_postural_diag], KP_postural_diag/1
  Demux1/2 -> KP_CoM_diag/1
  jointPos/1 -> STATE MACHINE/5(jointPos), xCom/2(jointPos), holder 2/1, xCom2/2(jointPos)
  fixed_l_sole_H_b/1 -> STATE MACHINE/9(l_sole_H_b), xCom/1(w_H_b)
  fixed_r_sole_H_b/1 -> xCom2/1(w_H_b), STATE MACHINE/10(r_sole_H_b)
  Clock1/1 -> STATE MACHINE/6(time)
  wrench_leftFoot/1 -> [wrench_leftFoot], STATE MACHINE/8(wrench_leftFoot)
  holder 1/1 -> STATE MACHINE/1(pos_CoM_0)
  holder 2/1 -> STATE MACHINE/2(jointPos_0)
  xCom2/1("pos_CoM_fixed_r_sole ") -> STATE MACHINE/4(pos_CoM_fixed_r_sole)
  STATE MACHINE/10(smoothingTimeCoM) -> smoothingTime_CoM/1
  STATE MACHINE/1(w_H_b) -> [w_H_b], w_H_b/1
  wrench_rightFoot/1 -> [wrench_rightFoot], STATE MACHINE/7(wrench_rightFoot)

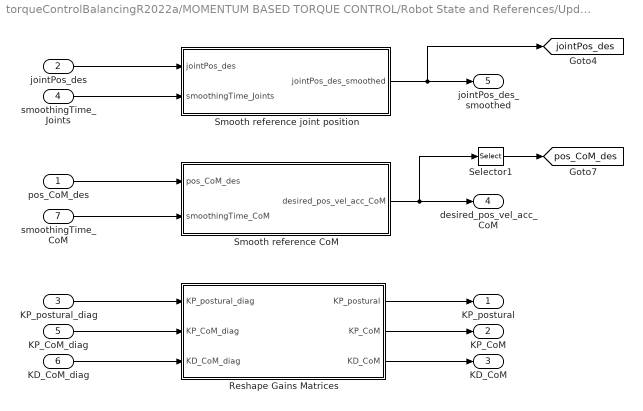
== system torqueControlBalancingR2022a/MOMENTUM BASED TORQUE CONTROL/Robot State and References/Update Gains and References ==
  pos_CoM_des : Inport
  jointPos_des : Inport  Port=2
  KP_postural_diag : Inport  Port=3
  smoothingTime_Joints : Inport  Port=4
  KP_CoM_diag : Inport  Port=5
  KD_CoM_diag : Inport  Port=6
  smoothingTime_CoM : Inport  Port=7
  Reshape Gains Matrices : Subsystem
  Selector1 : Selector  NumberOfDimensions=2  InputPortWidth=3  IndexOptions=Index vector (dialog),Index vector (dialog)  Indices=[1 2 3],[1]  OutputSizes=1,1
  Smooth reference CoM : Subsystem
  Smooth reference joint position : Subsystem
  KP_postural : Outport  VectorParamsAs1DForOutWhenUnconnected=off
  KP_CoM : Outport  Port=2  VectorParamsAs1DForOutWhenUnconnected=off
  KD_CoM : Outport  Port=3  VectorParamsAs1DForOutWhenUnconnected=off
  desired_pos_vel_acc_CoM : Outport  Port=4  VectorParamsAs1DForOutWhenUnconnected=off
  jointPos_des_smoothed : Outport  Port=5  VectorParamsAs1DForOutWhenUnconnected=off
  tag scope: jointPos_des=global, pos_CoM_des=global
  wires:
  Smooth reference joint position/1(jointPos_des_smoothed) -> [jointPos_des], jointPos_des_smoothed/1
  jointPos_des/1 -> Smooth reference joint position/1(jointPos_des)
  smoothingTime_Joints/1 -> Smooth reference joint position/2(smoothingTime_Joints)
  pos_CoM_des/1 -> Smooth reference CoM/1(pos_CoM_des)
  smoothingTime_CoM/1 -> Smooth reference CoM/2(smoothingTime_CoM)
  Smooth reference CoM/1(desired_pos_vel_acc_CoM) -> Selector1/1, desired_pos_vel_acc_CoM/1
  KP_postural_diag/1 -> Reshape Gains Matrices/1(KP_postural_diag)
  KP_CoM_diag/1 -> Reshape Gains Matrices/2(KP_CoM_diag)
  KD_CoM_diag/1 -> Reshape Gains Matrices/3(KD_CoM_diag)
  Reshape Gains Matrices/1(KP_postural) -> KP_postural/1
  Reshape Gains Matrices/2(KP_CoM) -> KP_CoM/1
  Reshape Gains Matrices/3(KD_CoM) -> KD_CoM/1
  Selector1/1 -> [pos_CoM_des]
